simulink model "Muscel_Model"  (R2016b)
settings: Solver=ode45  StartTime=0.0  StopTime=30  FixedStep=0.001  MinStep=0.0001  RelTol=1e-3
libraries: simulink x3
settings Model: Creator=Jan  LastModifiedBy=GuopingZhao

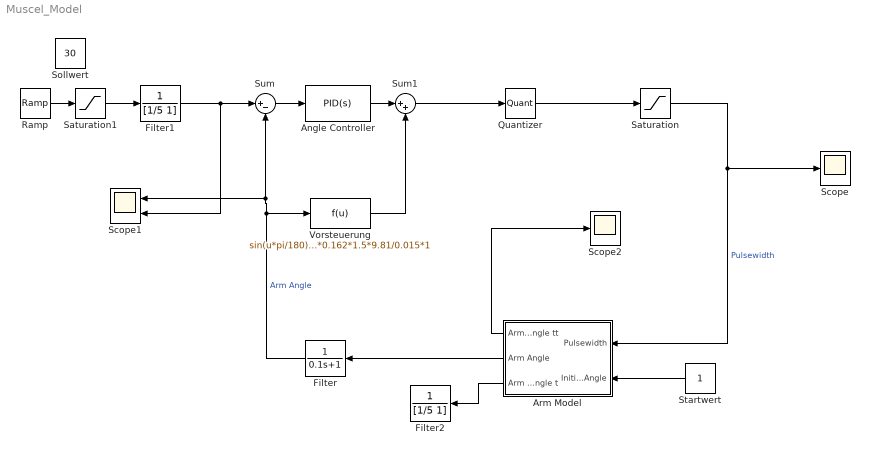
== system Muscel_Model ==
  Angle Controller : simulink/Continuous/PID Controller  Controller=PID  TimeDomain=Continuous-time  SampleTime=-1  IntegratorMethod=Forward Euler  FilterMethod=Forward Euler  Form=Parallel  UseFilter=on  ControllerParametersSource=internal  P=2  I=2  D=0  N=100  InitialConditionSource=internal  InitialConditionForIntegrator=0  InitialConditionForFilter=0  ExternalReset=none  LimitOutput=off  UpperSaturationLimit=500  LowerSaturationLimit=-inf  LinearizeAsGain=on  AntiWindupMode=none  Kb=1  TrackingMode=off  Kt=1  PParamMin=[]  PParamMax=[]  IParamMin=[]  IParamMax=[]  DParamMin=[]  DParamMax=[]  NParamMin=[]  NParamMax=[]  KbParamMin=[]  KbParamMax=[]  KtParamMin=[]  KtParamMax=[]  POutMin=[]  POutMax=[]  IOutMin=[]  IOutMax=[]  DOutMin=[]  DOutMax=[]  NOutMin=[]  NOutMax=[]  KbOutMin=[]  KbOutMax=[]  KtOutMin=[]  KtOutMax=[]  IntegratorOutMin=[]  IntegratorOutMax=[]  FilterOutMin=[]  FilterOutMax=[]  SumOutMin=[]  SumOutMax=[]  SumI1OutMin=[]  SumI1OutMax=[]  SumI2OutMin=[]  SumI2OutMax=[]  SumI3OutMin=[]  SumI3OutMax=[]  SumDOutMin=[]  SumDOutMax=[]  SaturationOutMin=[]  SaturationOutMax=[]  IntegratorContinuousStateAttributes=''  IntegratorStateMustResolveToSignalObject=off  IntegratorRTWStateStorageClass=Auto  FilterContinuousStateAttributes=''  FilterStateMustResolveToSignalObject=off  FilterRTWStateStorageClass=Auto  DifferentiatorICPrevScaledInput=0  DifferentiatorOutMin=[]  DifferentiatorOutMax=[]
  Arm Model : Subsystem
  Filter : TransferFcn  Denominator=[0.1 1]
  Filter1 : TransferFcn  Denominator=[1/5 1]
  Filter2 : TransferFcn  Denominator=[1/5 1]
  Quantizer : Quantizer  QuantizationInterval=10
  Ramp : simulink/Sources/Ramp  slope=5  start=1  X0=0
  Saturation : Saturate  UpperLimit=500  LowerLimit=0
  Saturation1 : Saturate  UpperLimit=30  LowerLimit=0
  Scope : Scope
  Scope1 : Scope  NumInputPorts=2
  Scope2 : Scope
  "Sollwert " : Constant  Value=30
  Startwert : Constant
  Sum : Sum  Inputs=|+-
  Sum1 : Sum  Inputs=|++
  Vorsteuerung : Fcn  Expr=sin(u*pi/180)*0.162*1.5*9.81/0.015*1
  wires:
  Sum/1 -> Angle Controller/1
  Quantizer/1 -> Saturation/1
  Startwert/1 -> Arm Model/2(Initial Angle)
  Saturation/1 -> Arm Model/1(Pulsewidth), Scope/1  "Pulsewidth"
  Angle Controller/1 -> Sum1/1
  Sum1/1 -> Quantizer/1
  Arm Model/2(Arm Angle) -> Filter/1
  Filter/1 -> Sum/2, Scope1/1, Vorsteuerung/1  "Arm Angle"
  Filter1/1 -> Scope1/2, Sum/1
  Arm Model/3(Arm Angle t) -> Filter2/1
  Arm Model/1(Arm Angle tt) -> Scope2/1
  Ramp/1 -> Saturation1/1
  Saturation1/1 -> Filter1/1
  Vorsteuerung/1 -> Sum1/2

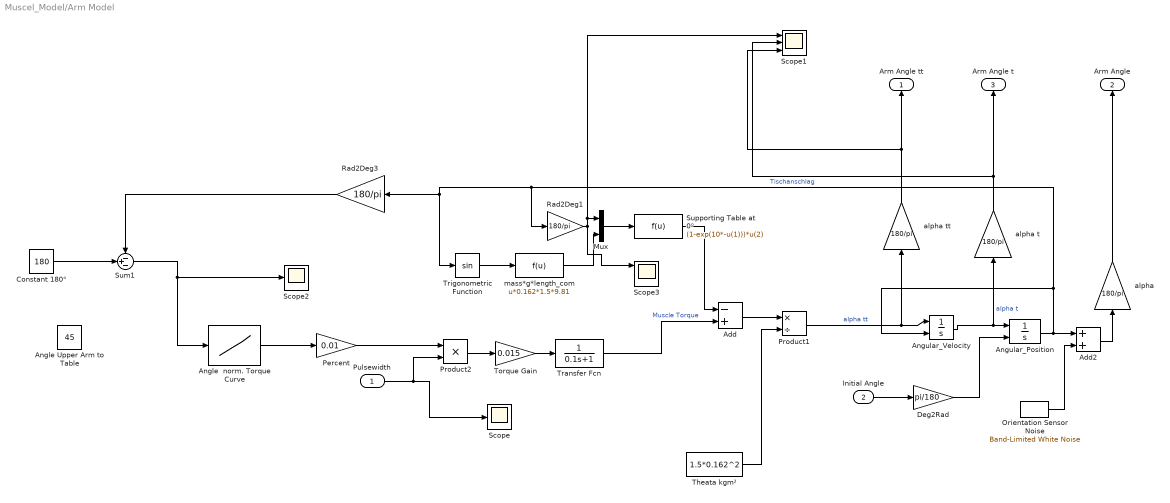
== system Muscel_Model/Arm Model ==
  Pulsewidth : Inport
  Initial Angle : Inport  Port=2
  Add : Sum  Inputs=-+
  Add2 : Sum
  Angle  norm. Torque Curve : Lookup_n-D  NumberOfTableDimensions=1  BreakpointsForDimension1=|  Table=|  InternalRulePriority=Speed  RndMeth=Simplest  InputSameDT=on
      BreakpointsForDimension1=|
      | [60.1
      | ;70.1;
      | 80.2;
      | 90.2;
      | 100.2;
      | 110.2
      | ;120.3;
      | 130.3;140.3
      | ;150.4;
      | 160.4]
      Table=|
      | [18;31;47;60;
      | 73;
      | 83
      | ;87;
      | 79;
      | 80;
      | 81
      | ;73]
  Angle Upper Arm to Table : Constant  Value=45
  Angular_Position : Integrator  InitialConditionSource=external  InitialCondition=45  LimitOutput=on  UpperSaturationLimit=90*pi/180  LowerSaturationLimit=0
  Angular_Velocity : Integrator  ExternalReset=falling
  Constant 180° : Constant  Value=180
  Deg2Rad : Gain  Gain=pi/180
  Mux : Mux  Inputs=2
  Orientation Sensor Noise : simulink/Sources/Band-Limited White Noise  Cov=[0.000001]  Ts=0.01  seed=[23341]
  Percent : Gain  Gain=0.01
  Product1 : Product  Inputs=*/
  Product2 : Product  Inputs=**
  Rad2Deg1 : Gain  Gain=180/pi
  Rad2Deg3 : Gain  Gain=180/pi
  Scope : Scope
  Scope1 : Scope  NumInputPorts=3
  Scope2 : Scope
  Scope3 : Scope  NumInputPorts=3
  Sum1 : Sum  Inputs=-+-
  Supporting Table at 0° : Fcn  Expr=(1-exp(10*-u(1)))*u(2)
  Theata kgm² : Constant  Value=1.5*0.162^2
  Torque Gain : Gain  Gain=0.015
  Transfer Fcn : TransferFcn  Denominator=[0.1 1]
  Trigonometric Function : Trigonometry
  alpha : Gain  Gain=180/pi
  alpha t : Gain  Gain=180/pi
  alpha tt : Gain  Gain=180/pi
  mass*g*length_com : Fcn  Expr=u*0.162*1.5*9.81
  Arm Angle tt : Outport
  Arm Angle : Outport  Port=2
  Arm Angle t : Outport  Port=3
  wires:
  Trigonometric Function/1 -> mass*g*length_com/1
  Angle  norm. Torque Curve/1 -> Percent/1
  Constant 180°/1 -> Sum1/2
  Sum1/1 -> Scope2/1, Angle  norm. Torque Curve/1
  Theata kgm²/1 -> Product1/2
  Angular_Velocity/1 -> alpha t/1, Angular_Position/1  "alpha t"
  Add/1 -> Product1/1
  Pulsewidth/1 -> Product2/2, Scope/1
  Percent/1 -> Product2/1
  Torque Gain/1 -> Transfer Fcn/1
  Product1/1 -> alpha tt/1, Angular_Velocity/1  "alpha tt"
  Angular_Position/1 -> Add2/1, Angular_Velocity/2, Rad2Deg1/1, Rad2Deg3/1, Trigonometric Function/1  "Tischanschlag"
  Deg2Rad/1 -> Angular_Position/2
  alpha tt/1 -> Scope1/3, Arm Angle tt/1
  Add2/1 -> alpha/1
  alpha/1 -> Arm Angle/1
  Rad2Deg3/1 -> Sum1/1
  Initial Angle/1 -> Deg2Rad/1
  Mux/1 -> Supporting Table at 0°/1
  Rad2Deg1/1 -> Scope3/1, Scope1/1, Mux/1
  Transfer Fcn/1 -> Add/2  "Muscle Torque"
  alpha t/1 -> Arm Angle t/1, Scope1/2
  Orientation Sensor Noise/1 -> Add2/2
  mass*g*length_com/1 -> Mux/2
  Supporting Table at 0°/1 -> Add/1
  Product2/1 -> Torque Gain/1
